simulink model "ATOM_simple_planning_simulator"  (R2026a)
settings: Solver=ode4  StopTime=50  FixedStep=0.01
StopFcn:
  | if exist('costmap_active','var') && ...
  |    exist('vehicle','var') && ...
  |    exist('parking_path','var') && ...
  |    ~isempty(parking_path)
  | 
  |     plotPlan(costmap_active, vehicle, parking_path);
  | else
  |     warning('No valid parking path is available for plotting.');
  | end
model workspace (MAT data in the model file):
  vehicle : object (value not decoded)
symbols that are objects in the model workspace (value not decoded): vehicle
undefined symbols (not defined in the file or in its folder): delta_f_LUT, gain4WS_LUT, k_ref_LUT, kappa_gain_BP, Ki, Kp, lateral, longitudinal, planning_validator, rr_gain_BP, rr_LUT, stanley, velocity_smoother
libraries: slpidlib x1, simulink x1
(part 5 of 7)

== matlab function ATOM_simple_planning_simulator/Plot vehicle/Plot vehicle Front reference frame ==
  settings: updateMethod=DISCRETE
  data: kinematic input Bus: KinematicStateBus; steer_front input double; steer_rear input double; veh input; traj input
function plotVehicleFront(kinematic, steer_front, steer_rear, veh, traj)

%% Vehicle parameters

L  = veh(3);
track = veh(4);

front_overhang = veh(5);
rear_overhang  = veh(6);
left_overhang = veh(7);
right_overhang = veh(8);

vehicle_length  = L + front_overhang + rear_overhang;
vehicle_width = track + left_overhang + right_overhang;

wheel_width = veh(2);
wheel_radius = veh(1);

%% Reference trajectory

x_ref = traj.pose.position.x;
y_ref = traj.pose.position.y;

yaw_ref = zeros(length(x_ref),1);


for i=1:length(x_ref)

    yaw_ref(i)=2*atan2(...
        traj.pose.orientation.qz(i),...
        traj.pose.orientation.qw(i));
end


%% Current kinematic state

x = kinematic.pose.position.x;
y = kinematic.pose.position.y;

qz = kinematic.pose.orientation.z;
qw = kinematic.pose.orientation.w;

yaw = 2*atan2(qz,qw);

vx = kinematic.twist.linear.x;

steer_front = steer_front;
steer_rear = steer_rear;

%% Position and orientation vehicle body

vehicle_body = [front_overhang vehicle_width/2;
                front_overhang -vehicle_width/2;
                -L-rear_overhang -vehicle_width/2;
                -L-rear_overhang vehicle_width/2;
                front_overhang vehicle_width/2];

R_body = [ cos(yaw) -sin(yaw)
    sin(yaw)  cos(yaw) ];

body_world = (R_body*vehicle_body')';

body_world(:,1)=body_world(:,1)+x;
body_world(:,2)=body_world(:,2)+y;


%% Position and orientation wheels

wheel_body = [wheel_radius  wheel_width/2
                wheel_radius -wheel_width/2
                -wheel_radius -wheel_width/2
                -wheel_radius  wheel_width/2
                wheel_radius  wheel_width/2];

FL = [0  track/2];
FR = [0 -track/2];
RL = [-L  track/2];
RR = [-L -track/2];

centers = [FL;
    FR;
    RL;
    RR];

centers = (R_body*centers')';

centers(:,1) = centers(:,1)+x;
centers(:,2) = centers(:,2)+y;

wheelFL = transformWheel(centers(1,:),steer_front,yaw,wheel_body);
wheelFR = transformWheel(centers(2,:),steer_front,yaw,wheel_body);
wheelRL = transformWheel(centers(3,:),steer_rear,yaw,wheel_body);
wheelRR = transformWheel(centers(4,:),steer_rear,yaw,wheel_body);



persistent hFig
persistent ax
persistent hBody
persistent hWheelFL
persistent hWheelFR
persistent hWheelRL
persistent hWheelRR
persistent hTrajectory
persistent TrajX
persistent TrajY
persistent hRefTraj 
persistent hArrow


if isempty(hBody)
    hFig = figure(13);
    clf

    ax = axes(hFig);

    hold(ax,'on')
    axis(ax,'equal')
    grid(ax,'on')


    xlabel(ax,'x [m]')
    ylabel(ax,'y [m]')

    hBody = plot(body_world(:,1),...
        body_world(:,2),...
        'k','LineWidth',2);

    hWheelFL = plot(wheelFL(:,1),...
        wheelFL(:,2),...
        'r','LineWidth',2);

    hWheelFR = plot(wheelFR(:,1),...
        wheelFR(:,2),...
        'r','LineWidth',2);

    hWheelRL = plot(wheelRL(:,1),...
        wheelRL(:,2),...
        'b','LineWidth',2);

    hWheelRR = plot(wheelRR(:,1),...
        wheelRR(:,2),...
        'b','LineWidth',2);

    TrajX = x;
    TrajY = y;

    hTrajectory = plot(TrajX,...
                       TrajY,...
                       'g','LineWidth',1);

    hRefTraj=plot(x_ref,y_ref,'b','LineWidth',2);

    step=5;

    hArrow=quiver(...
        x_ref(1:step:end),...
        y_ref(1:step:end),...
        cos(yaw_ref(1:step:end)),...
        sin(yaw_ref(1:step:end)),...
        0.5,...
        'r');

else

    set(hBody,...
        'XData',body_world(:,1),...
        'YData',body_world(:,2));

    set(hWheelFL,...
        'XData',wheelFL(:,1),...
        'YData',wheelFL(:,2));

    set(hWheelFR,...
        'XData',wheelFR(:,1),...
        'YData',wheelFR(:,2));

    set(hWheelRL,...
        'XData',wheelRL(:,1),...
        'YData',wheelRL(:,2));

    set(hWheelRR,...
        'XData',wheelRR(:,1),...
        'YData',wheelRR(:,2));

    TrajX(end+1) = x;
    TrajY(end+1) = y;

 
    set(hTrajectory,...
        'XData',TrajX,...
        'YData',TrajY);

    set(hRefTraj,...
        'XData',x_ref,...
        'YData',y_ref);

    

end

margin = 12;
xlim(ax, [x-margin x+margin])
ylim(ax, [y-margin y+margin])

% xlim([-20 20])
% ylim([-20 20])

drawnow limitrate
pause(0.01)


end

== matlab function ATOM_simple_planning_simulator/Plot vehicle/SetStanleyTrajectory/calcLongOffsetToSegment ==
  data: seg_idx input; ego_pose input; trajectory input Bus: TrajectoryDataBus; ego_offset_to_segment output
function ego_offset_to_segment = calcLongOffsetToSegment(seg_idx, ego_pose, trajectory)

ego_offset_to_segment = calcLongitudinalOffsetToSegment(trajectory, seg_idx, ego_pose);

end

== matlab function ATOM_simple_planning_simulator/Plot vehicle/SetStanleyTrajectory/findFirstNearestSegmentIndexWithSoftConstraints ==
  data: trajectory input; dist_threshold input; yaw_threshold input; nearest_seg_idx output; pose input
function nearest_seg_idx = findNearestSegmentIndexWithSoftConstraints( ...
    trajectory, dist_threshold, yaw_threshold, pose)


%% Step 1:
% Find nearest point index

nearest_idx = findFirstNearestIndexWithSoftConstraints( ...
    trajectory, ...
    pose, ...
    dist_threshold, ...
    yaw_threshold);


N = length(trajectory.pose.position.x);


%% Step 2:
% Convert point index into segment index

% First point
if nearest_idx == 1

    nearest_seg_idx = 1;
    return

end


% Last point
if nearest_idx == N

    nearest_seg_idx = N-1;
    return

end



%% Step 3:
% Determine whether ego lies before or after nearest point
%
% Equivalent to Autoware:
%
% signed_length =
% calcLongitudinalOffsetToSegment(points,
%                                 nearest_idx,
%                                 pose.position)


signed_length = calcLongitudinalOffsetToSegment( ...
    trajectory,...
    nearest_idx,...
    pose);



%% Step 4:
% Choose segment

if signed_length <= 0

    % ego is before nearest point
    %
    % Autoware:
    % return nearest_idx - 1;

    nearest_seg_idx = nearest_idx - 1;


else

    % ego is after nearest point
    %
    % Autoware:
    % return nearest_idx;

    nearest_seg_idx = nearest_idx;

end


end

== matlab function ATOM_simple_planning_simulator/Lateral run()/CalculateStanley/getData/calculate curvature predicted/CalcTrajectoryCurvature ==
  data: trajectory input Bus: TrajectoryDataBus; curvature output; nearest_idx input; idx_dist input
function curvature = ComputeNearestCurvature( ...
    trajectory,...
    nearest_idx, idx_dist)


%% ============================================================
% COMPUTE NEAREST TRAJECTORY CURVATURE
%
% Equivalent to:
%
% autoware::motion_utils::calcTrajectoryCurvatureFrom3Points()
%
% Difference:
%
% - Autoware computes curvature for the whole trajectory
% - Here only the curvature at nearest_idx is required
%   for Stanley controller
%
% Inputs:
%
% trajectory:
%   Reference trajectory
%
% nearest_idx:
%   Nearest trajectory point index
%
% idx_dist:
%   Distance in samples used for three-point fitting
%
%
% Output:
%
% curvature:
%   Local trajectory curvature [1/m]
%
% ============================================================

N = length(trajectory.pose.position.x);



%% Check trajectory length

if N < 3

    curvature = 0;
    return

end



%% Clamp index

nearest_idx = max(1,min(nearest_idx,N));



%% Select three points
%
% Equivalent to Autoware:
%
% p0 = trajectory[i-idx_dist]
% p1 = trajectory[i]
% p2 = trajectory[i+idx_dist]
%
% ============================================================


idx_prev = nearest_idx - min(idx_dist, nearest_idx-1);

idx_next = nearest_idx + min(idx_dist, N-nearest_idx);



p0 = [
    trajectory.pose.position.x(idx_prev),...
    trajectory.pose.position.y(idx_prev)
];


p1 = [
    trajectory.pose.position.x(nearest_idx),...
    trajectory.pose.position.y(nearest_idx)
];


p2 = [
    trajectory.pose.position.x(idx_next),...
    trajectory.pose.position.y(idx_next)
];



%% Compute curvature

curvature = calc_curvature(p0,p1,p2);


end

== matlab function ATOM_simple_planning_simulator/Lateral run()/CalculateStanley/getData/calculate curvature predicted/ComputeIdxDist ==
  data: points_interval input; idx_dist output; vel_smoother input
function idx_dist = ComputeIdxDist( ...
    points_interval, ...
    vel_smoother)

% ComputeIdxDist
%
% Computes the point offset used for trajectory curvature estimation.
%
% The curvature is evaluated using three trajectory points separated by a
% fixed physical distance. Since the trajectory is sampled with a constant
% spatial interval (points_interval), this function converts the desired
% curvature calculation distance into the corresponding point index offset.
%
% In other words, idx_dist represents the number of trajectory points
% corresponding to the specified curvature calculation distance.
%
% Equivalent to the Autoware implementation:
%
% idx_dist = max(int(curvature_calculation_distance / points_interval), 1);

curvature_calculation_distance = vel_smoother(1);

idx_dist = max( ...
    floor(curvature_calculation_distance / points_interval), ...
    1);

== matlab function ATOM_simple_planning_simulator/Lateral run()/CalculateStanley/getData/calculate curvature predicted/ComputePointsInterval ==
  data: input_points_interval input; vel_smoother input; use_resampling input; points_interval output
function points_interval = computePointsInterval(input_points_interval, ...
    vel_smoother, use_resampling)

% Compute the trajectory points interval used for preprocessing.
%
% If resampling is enabled, a constant spatial interval is imposed.
% Otherwise, the original trajectory point spacing is preserved.

sample_ds = vel_smoother(3,1);

if use_resampling

    points_interval = sample_ds;

else

    points_interval = input_points_interval;

end

end

== matlab function ATOM_simple_planning_simulator/Lateral run()/CalculateStanley/VerifyStanleyStatus ==
  data: steering_cmd input; stanley_solved_status output boolean; reason output
function [stanley_solved_status, reason] = VerifyStanleyStatus(steering_cmd)

% reason codes:
% 0 = OK
% 1 = Steering command is NaN/Inf
%
% Attention: in Autoware, reason is a String type. Just Simulink struggles
% with it.

stanley_solved_status = true;
reason = uint8(0);

if ~isfinite(steering_cmd)
    stanley_solved_status = false;
    reason = uint8(1);
end

== matlab function ATOM_simple_planning_simulator/Lateral run()/MATLAB Function1 ==
  data: solved input; previous_status output; reason input; previous_status input; previous_reason input; previous_reason output
function [previous_status, previous_reason] = StanleyStatusManager( ...
    solved,...
    reason,...
    previous_status,...
    previous_reason)

% ATTENTION!!!
% In Autoware, stanley_solved_status (originally mpc_solved_status) 
% is a struct, where equivalently:
% - solved = stanley_solved_status.result
% - reason = stanley_solved_status.reason
%
% StanleyStatusManager here is not implemented since it doesn't change the
% implementation of the controller.

previous_status = solved;
previous_reason = reason;

== matlab function ATOM_simple_planning_simulator/Parking Scenario/Costmap generation: perpendicular lot/Perpendicular Parking ==
  settings: updateMethod=DISCRETE
  data: veh input; costmap output Bus: OccupancyGridBus; start_pose output; goal_pose output
function [costmap, start_pose, goal_pose] = costmapPerpendicularLot(veh)
%COSTMAPPERPENDICULARLOT  Single row of 7 bays, one left empty at x = 0.
%
% Reproduces autoware_costmap_generator geometry:
%   grid_resolution 0.3, grid_length_x/y 70.0, expand_polygon_size 0.5
% The primitives layer is INVERTED: background occupied, lot carved out.

persistent occ

res = 0.3;   W = 234;   H = 234;
origin_x = -(W/2)*res;
origin_y = -(H/2)*res;

bay_x     = (-3:3)*3.6;      % 7 bays, 3.6 m pitch
bay_y     = 8.75;
empty_bay = 4;               % x = 0

if isempty(occ)
    [IX, IY] = meshgrid(0:W-1, 0:H-1);
    X = origin_x + IX*res;
    Y = origin_y + IY*res;

    lot_x = [-15  15  15 -15];
    lot_y = [-12 -12  12  12];
    occ = ones(H,W);
    occ(inpolygon(X, Y, lot_x, lot_y)) = 0;

    car_len = veh(5) + veh(3) + veh(6);
    car_wid = veh(4) + veh(7) + veh(8);
    expand  = 0.5;
    L = car_len + expand;
    D = car_wid + expand;

    for k = 1:7
        if k ~= empty_bay
            qx = [ D/2 -D/2 -D/2  D/2] + bay_x(k);
            qy = [ L/2  L/2 -L/2 -L/2] + bay_y;
            occ(inpolygon(X, Y, qx, qy)) = 1;
        end
    end
end

start_pose = [0, 0,    0];
goal_pose  = [0, 7.75, pi/2];

costmap.info.resolution           = res;
costmap.info.width                = uint32(W);
costmap.info.height               = uint32(H);
costmap.info.origin.position.x    = origin_x;
costmap.info.origin.position.y    = origin_y;
costmap.info.origin.position.z    = 0;
costmap.info.origin.orientation.x = 0;
costmap.info.origin.orientation.y = 0;
costmap.info.origin.orientation.z = 0;
costmap.info.origin.orientation.w = 1;
costmap.data                      = int8(occ*100);
end

== matlab function ATOM_simple_planning_simulator/Lateral run()/UpdateSteeringOffset ==
  settings: updateMethod=DISCRETE
  data: steering input; twist input Bus: TwistBus; wheel_base input; update_vel_threshold input; update_steer_threshold input; average_num input; offset_limit input; steering_offset output; veh input
function steering_offset = updateSteeringOffset( ...
    steering,...
    twist,...
    wheel_base,...
    update_vel_threshold,...
    update_steer_threshold,...
    average_num,...
    offset_limit, ...
    veh)


persistent offset_storage
persistent count
persistent current_offset

rear_steering_ratio = veh(29);

if isempty(offset_storage)

    offset_storage = zeros(average_num,1);
    count = 0;
    current_offset = 0;

end


%% Current vehicle state

vx = twist.linear.x;
yaw_rate = twist.angular.z;



%% Check if offset update is allowed

update_offset = ...
    abs(vx) > update_vel_threshold && ...
    abs(steering) < update_steer_threshold;



if update_offset


    %% Estimate steering from vehicle motion

    rear_steering = rear_steering_ratio * steering;

    steer_angle_est = atan( ...
        yaw_rate*wheel_base/vx + tan(rear_steering));



    %% Compute offset

    new_offset = steering - steer_angle_est;



    %% Circular buffer

    count = count + 1;


    if count <= average_num

        offset_storage(count) = new_offset;

    else

        % shift left

        offset_storage(1:end-1)=offset_storage(2:end);

        offset_storage(end)=new_offset;

    end



    %% Compute average

    valid_samples = min(count,average_num);

    current_offset = mean(offset_storage(1:valid_samples));


end



%% Saturation (Autoware getOffset)

steering_offset = min(max(current_offset,...
    -offset_limit),...
    offset_limit);

end

== matlab function ATOM_simple_planning_simulator/Lateral run()/CalculateStanley/getData/calcNearestPoseInterpStanley1 ==
  data: self_pose input Bus: KinematicStateBus; trajectory input Bus: TrajectoryDataBus; nearest_pose output Bus: PoseBusStanley; max_dist input; max_yaw input; nearest_idx output
function [nearest_pose,nearest_idx]  = calcNearestPoseInterpStanley( ...
    self_pose, ...
    trajectory, ...
    max_dist, ...
    max_yaw)


%% ============================================================
% CALC NEAREST POSE INTERPOLATION FOR STANLEY CONTROLLER
%
% Equivalent to:
%
% MPCUtils::calcNearestPoseInterp()
%
% Differences with MPC:
%
% - Input trajectory is directly Trajectory message
% - No MPCTrajectory conversion
% - No relative_time prediction
% - Reference is already transformed to FRONT AXLE
%
% The function returns the continuous closest pose of the
% front axle on the reference trajectory.
%
% ============================================================


N = length(trajectory.pose.position.x);



%% ============================================================
% Initialization for code generation
% ============================================================

nearest_pose = struct();

nearest_pose.position.x = 0;
nearest_pose.position.y = 0;
nearest_pose.orientation.x = 0;
nearest_pose.orientation.y = 0;
nearest_pose.orientation.z = 0;
nearest_pose.orientation.w = 0;

nearest_idx = 1;

% nearest_velocity = 0;



if N == 0

    return

end



%% ============================================================
% Step 1:
% Find nearest trajectory index
%
% Equivalent to:
%
% findFirstNearestIndexWithSoftConstraints()
%
% ============================================================


nearest_idx = findFirstNearestIndexWithSoftConstraints( ...
    trajectory,...
    self_pose,...
    max_dist,...
    max_yaw);



%% ============================================================
% Single point trajectory
%
% Equivalent Autoware:
%
% if traj.size()==1
%
% ============================================================


if N == 1

    nearest_pose.x = trajectory.pose.position.x(1);
    nearest_pose.y = trajectory.pose.position.y(1);

    nearest_pose.orientation.x = trajectory.pose.orientation.qx(1);
    nearest_pose.orientation.y = trajectory.pose.orientation.qy(1);
    nearest_pose.orientation.z = trajectory.pose.orientation.qz(1);
    nearest_pose.orientation.w = trajectory.pose.orientation.qw(1);

    % nearest_velocity = trajectory.longitudinal_velocity_mps(1);

    return

end



%% ============================================================
% Step 2:
% Determine interpolation segment
%
% Equivalent to:
%
% calcLongitudinalOffset()
%
% ============================================================


if nearest_idx == 1

    prev_idx = 1;
    next_idx = 2;


elseif nearest_idx == N

    prev_idx = N-1;
    next_idx = N;


else


    p_nearest = [
        trajectory.pose.position.x(nearest_idx)
        trajectory.pose.position.y(nearest_idx)
        ];


    p_next = [
        trajectory.pose.position.x(nearest_idx+1)
        trajectory.pose.position.y(nearest_idx+1)
        ];


    signed_length = calcLongitudinalOffset( ...
        p_nearest,...
        p_next,...
        [self_pose.pose.position.x self_pose.pose.position.y]');


    if signed_length <= 0

        prev_idx = nearest_idx-1;
        next_idx = nearest_idx;

    else

        prev_idx = nearest_idx;
        next_idx = nearest_idx+1;

    end

end



%% ============================================================
% Step 3:
% Linear interpolation
%
% Equivalent to:
%
% nearest_pose.position =
% (1-ratio)*prev + ratio*next
%
% ============================================================


p_prev = [
    trajectory.pose.position.x(prev_idx)
    trajectory.pose.position.y(prev_idx)
];


p_next = [
    trajectory.pose.position.x(next_idx)
    trajectory.pose.position.y(next_idx)
];



segment_length = norm(p_next-p_prev);



% avoid division by zero

if segment_length < 1e-5


    nearest_pose.position.x = trajectory.pose.position.x(nearest_idx);
    nearest_pose.position.y = trajectory.pose.position.y(nearest_idx);


    nearest_pose.orientation.x = trajectory.pose.orientation.qx(nearest_idx);
    nearest_pose.orientation.y = trajectory.pose.orientation.qy(nearest_idx);
    nearest_pose.orientation.z = trajectory.pose.orientation.qz(nearest_idx);
    nearest_pose.orientation.w = trajectory.pose.orientation.qw(nearest_idx);

    % nearest_velocity = trajectory.longitudinal_velocity_mps(nearest_idx);


    return

end



%% Projection of ego on segment

offset = calcLongitudinalOffset( ...
    p_prev,...
    p_next,...
    [self_pose.pose.position.x self_pose.pose.position.y]');


ratio = min(max(offset / segment_length,0),1);



%% Interpolated position

nearest_pose.position.x = ...
    (1-ratio)*p_prev(1)+ratio*p_next(1);


nearest_pose.position.y = ...
    (1-ratio)*p_prev(2)+ratio*p_next(2);



%% ============================================================
% Yaw interpolation
%
% Equivalent:
%
% normalize_radian()
%
% ============================================================


yaw_prev = QuaternionToYaw( ...
    trajectory.pose.orientation.qx(prev_idx),...
    trajectory.pose.orientation.qy(prev_idx),...
    trajectory.pose.orientation.qz(prev_idx),...
    trajectory.pose.orientation.qw(prev_idx));


yaw_next = QuaternionToYaw( ...
    trajectory.pose.orientation.qx(next_idx),...
    trajectory.pose.orientation.qy(next_idx),...
    trajectory.pose.orientation.qz(next_idx),...
    trajectory.pose.orientation.qw(next_idx));


yaw_error = wrapToPi(yaw_prev-yaw_next);


nearest_yaw = wrapToPi( ...
    yaw_next + (1-ratio)*yaw_error);

[qx,qy,qz,qw] = yawToQuaternion(nearest_yaw);

nearest_pose.orientation.x = qx;
nearest_pose.orientation.y = qy;
nearest_pose.orientation.z = qz;
nearest_pose.orientation.w = qw;



% %% ============================================================
% % Velocity interpolation
% %
% % Stanley adaptation:
% %
% % The velocity is used for:
% % - gain scheduling
% % - softening factor
% %
% % ============================================================
% 
% 
% v_prev = trajectory.longitudinal_velocity_mps(prev_idx);
% 
% v_next = trajectory.longitudinal_velocity_mps(next_idx);
% 
% 
% nearest_velocity = ...
%     (1-ratio)*v_prev + ratio*v_next;


end

== matlab function ATOM_simple_planning_simulator/Lateral run()/CalculateStanley/getData/calculate curvature current/CalcTrajectoryCurvature ==
  data: trajectory input Bus: TrajectoryDataBus; curvature output; nearest_idx input; idx_dist input
function curvature = ComputeNearestCurvature( ...
    trajectory,...
    nearest_idx, idx_dist)


%% ============================================================
% COMPUTE NEAREST TRAJECTORY CURVATURE
%
% Equivalent to:
%
% autoware::motion_utils::calcTrajectoryCurvatureFrom3Points()
%
% Difference:
%
% - Autoware computes curvature for the whole trajectory
% - Here only the curvature at nearest_idx is required
%   for Stanley controller
%
% Inputs:
%
% trajectory:
%   Reference trajectory
%
% nearest_idx:
%   Nearest trajectory point index
%
% idx_dist:
%   Distance in samples used for three-point fitting
%
%
% Output:
%
% curvature:
%   Local trajectory curvature [1/m]
%
% ============================================================

N = length(trajectory.pose.position.x);



%% Check trajectory length

if N < 3

    curvature = 0;
    return

end



%% Clamp index

nearest_idx = max(1,min(nearest_idx,N));



%% Select three points
%
% Equivalent to Autoware:
%
% p0 = trajectory[i-idx_dist]
% p1 = trajectory[i]
% p2 = trajectory[i+idx_dist]
%
% ============================================================


idx_prev = nearest_idx - min(idx_dist, nearest_idx-1);

idx_next = nearest_idx + min(idx_dist, N-nearest_idx);



p0 = [
    trajectory.pose.position.x(idx_prev),...
    trajectory.pose.position.y(idx_prev)
];


p1 = [
    trajectory.pose.position.x(nearest_idx),...
    trajectory.pose.position.y(nearest_idx)
];


p2 = [
    trajectory.pose.position.x(idx_next),...
    trajectory.pose.position.y(idx_next)
];



%% Compute curvature

curvature = calc_curvature(p0,p1,p2);


end

== matlab function ATOM_simple_planning_simulator/Lateral run()/CalculateStanley/getData/calculate curvature current/ComputeIdxDist ==
  data: points_interval input; idx_dist output; vel_smoother input
function idx_dist = ComputeIdxDist( ...
    points_interval, ...
    vel_smoother)

% ComputeIdxDist
%
% Computes the point offset used for trajectory curvature estimation.
%
% The curvature is evaluated using three trajectory points separated by a
% fixed physical distance. Since the trajectory is sampled with a constant
% spatial interval (points_interval), this function converts the desired
% curvature calculation distance into the corresponding point index offset.
%
% In other words, idx_dist represents the number of trajectory points
% corresponding to the specified curvature calculation distance.
%
% Equivalent to the Autoware implementation:
%
% idx_dist = max(int(curvature_calculation_distance / points_interval), 1);

curvature_calculation_distance = vel_smoother(1);

idx_dist = max( ...
    floor(curvature_calculation_distance / points_interval), ...
    1);

== matlab function ATOM_simple_planning_simulator/Lateral run()/CalculateStanley/getData/calculate curvature current/ComputePointsInterval ==
  data: input_points_interval input; vel_smoother input; use_resampling input; points_interval output
function points_interval = computePointsInterval(input_points_interval, ...
    vel_smoother, use_resampling)

% Compute the trajectory points interval used for preprocessing.
%
% If resampling is enabled, a constant spatial interval is imposed.
% Otherwise, the original trajectory point spacing is preserved.

sample_ds = vel_smoother(3,1);

if use_resampling

    points_interval = sample_ds;

else

    points_interval = input_points_interval;

end

end

== matlab function ATOM_simple_planning_simulator/Lateral run()/CalculateStanley/RearToFrontOdometry ==
  data: rear_pose input Bus: KinematicStateBus; front_pose_pred output Bus: KinematicStateBus; wheel_base input
function front_pose_pred = RearToFrontOdometryCurrent( ...
    rear_pose, ...
    wheel_base)

front_pose_pred = rear_pose;

% 1. Estrazione dello Yaw dall'orientamento (Quaternion -> Yaw)
qx = rear_pose.pose.orientation.x;
qy = rear_pose.pose.orientation.y;
qz = rear_pose.pose.orientation.z;
qw = rear_pose.pose.orientation.w;
yaw = QuaternionToYaw(qx, qy, qz, qw);

% 2. Calcolo della Posizione Attuale dell'Asse Anteriore (Mappa/World Frame)
x_front_now = rear_pose.pose.position.x + wheel_base * cos(yaw);
y_front_now = rear_pose.pose.position.y + wheel_base * sin(yaw);

% 3. Velocità dell'Asse Anteriore espresso nel Frame Veicolo (Body Frame)
v_x_body = rear_pose.twist.linear.x;
v_y_body = rear_pose.twist.linear.y + rear_pose.twist.angular.z * wheel_base;

% 4. Conversione delle Velocità dal Frame Veicolo (Body) al Frame Mappa (World)
% Ruotiamo il vettore velocità [v_x_body, v_y_body] dell'angolo yaw attuale:
v_x_world = v_x_body * cos(yaw) - v_y_body * sin(yaw);
v_y_world = v_x_body * sin(yaw) + v_y_body * cos(yaw);

% 5. PREDIZIONE TEMPORALE (Coordinate t + tau nel Frame Mappa)
front_pose_pred.pose.position.x = x_front_now;
front_pose_pred.pose.position.y = y_front_now;
front_pose_pred.pose.position.z = rear_pose.pose.position.z;

% 6. Aggiornamento delle velocità nel messaggio di output (Frame Veicolo)
front_pose_pred.twist.linear.x = v_x_body;
front_pose_pred.twist.linear.y = v_y_body;
front_pose_pred.twist.linear.z = rear_pose.twist.linear.z;

% 7. L'orientamento rimane lo stesso (o aggiornato con il pitch/roll se presente)
front_pose_pred.pose.orientation = rear_pose.pose.orientation;

end

== matlab function ATOM_simple_planning_simulator/Lateral run()/CalculateStanley/getData/ChooseCurvature ==
  data: curvature_pred input; curvature output; curvature_curr input
function curvature = ChooseCurvature(curvature_pred, curvature_curr)

% =========================================
%
% Left turns: curvature > 0
% Right turns: curvature < 0
%
% =========================================

curvature_max = sin(2*0.7)/(2*cos(-0.7));

if abs(curvature_pred) >= abs(curvature_curr)
    if abs(curvature_pred) >= curvature_max
        sign_k = sign(curvature_pred);
        curvature = sign_k*curvature_max;
    else
        curvature = curvature_pred;
    end
else
    if abs(curvature_curr) >= curvature_max
        sign_k = sign(curvature_curr);
        curvature = sign_k*curvature_max;
    else
        curvature = curvature_curr;
    end


end

== matlab function ATOM_simple_planning_simulator/Lateral run()/Adaptive d0 ==
  data: d0 output; tau_steer input
function d0 = ComputeAdaptived0(tau_steer)

% d0 is the distance ahead of the vehicle, necessary for prediction.
% It's independent from current vehicle speed.
% We've seen that with time_constant = 0.27 --> d0 = 0.3.

d0 = (0.3/0.27)*tau_steer;

end

== matlab function ATOM_simple_planning_simulator/Lane Follower Scenario/Demanded trajectory generation: Serpentine/Trajectory Generator: 90° left turn critical for 2WS ==
  data: x output; y output; z output; qx output; qy output; qz output; qw output; longitudinal_velocity_mps output; lateral_velocity_mps output; acceleration_mps2 output; heading_rate_rps output; front_wheel_angle_rad output; rear_wheel_angle_rad output
function [x,y,z,qx,qy,qz,qw,...
          longitudinal_velocity_mps,...
          lateral_velocity_mps,...
          acceleration_mps2,...
          heading_rate_rps,...
          front_wheel_angle_rad,...
          rear_wheel_angle_rad] = trajectoryGenerator

N = 100;

%% Geometry

R = 3;                  % Radius [m]

N1 = 20;                % First straight
N2 = 30;                % Left curve
N3 = 30;                % Right curve
N4 = 20;                % Final straight


%% Allocate outputs

x = zeros(N,1);
y = zeros(N,1);
z = zeros(N,1);

qx = zeros(N,1);
qy = zeros(N,1);
qz = zeros(N,1);
qw = zeros(N,1);

longitudinal_velocity_mps = 6/3.6 * ones(N,1);

lateral_velocity_mps = zeros(N,1);
acceleration_mps2 = zeros(N,1);
heading_rate_rps = zeros(N,1);

front_wheel_angle_rad = zeros(N,1);
rear_wheel_angle_rad = zeros(N,1);


%% ========================================================================
%% First straight
%% ========================================================================

L1 = 2;

for i = 1:N1

    t = (i-1)/(N1-1);

    x(i) = t*L1;
    y(i) = 0;

    yaw = 0;

    qz(i) = sin(yaw/2);
    qw(i) = cos(yaw/2);

end


%% ========================================================================
%% First curve (LEFT)
%% ========================================================================

center1_x = L1;
center1_y = R;

theta = linspace(-pi/2,0,N2);

for k = 1:N2

    i = N1 + k;

    x(i) = center1_x + R*cos(theta(k));
    y(i) = center1_y + R*sin(theta(k));

    yaw = theta(k) + pi/2;

    qz(i) = sin(yaw/2);
    qw(i) = cos(yaw/2);

end


%% ========================================================================
%% Second curve (RIGHT)
%% Tangent to the previous one
%% ========================================================================

x_join = x(N1+N2);
y_join = y(N1+N2);

center2_x = x_join + R;
center2_y = y_join;

theta = linspace(pi,pi/2,N3);

for k = 1:N3

    i = N1 + N2 + k;

    x(i) = center2_x + R*cos(theta(k));
    y(i) = center2_y + R*sin(theta(k));

    yaw = theta(k) - pi/2;

    qz(i) = sin(yaw/2);
    qw(i) = cos(yaw/2);

end


%% ========================================================================
%% Final straight
%% ========================================================================

L2 = 15;

x0 = x(N1+N2+N3);
y0 = y(N1+N2+N3);

for k = 1:N4

    i = N1 + N2 + N3 + k;

    t = k/N4;

    x(i) = x0 + t*L2;
    y(i) = y0;

    yaw = 0;

    qz(i) = sin(yaw/2);
    qw(i) = cos(yaw/2);

end

end

== matlab function ATOM_simple_planning_simulator/Lane Follower Scenario/Demanded trajectory generation: smooth Parabola/Smoothed Parabola trajectory ==
  data: x output double; y output double; z output double; qx output double; qy output double; qz output double; qw output double; longitudinal_velocity_mps output double; lateral_velocity_mps output; acceleration_mps2 output; heading_rate_rps output; front_wheel_angle_rad output; rear_wheel_angle_rad output
function [x,y,z,qx,qy,qz,qw,longitudinal_velocity_mps, lateral_velocity_mps, acceleration_mps2, heading_rate_rps, front_wheel_angle_rad, rear_wheel_angle_rad] ...
            = trajectoryGenerator

N=100;

L=50;
Yend=20;


x=zeros(N,1);
y=zeros(N,1);
z=zeros(N,1);


qx=zeros(N,1);
qy=zeros(N,1);
qz=zeros(N,1);
qw=zeros(N,1);

longitudinal_velocity_mps=zeros(N,1);
lateral_velocity_mps=zeros(N,1);
acceleration_mps2=zeros(N,1);
heading_rate_rps=zeros(N,1);
front_wheel_angle_rad=zeros(N,1);
rear_wheel_angle_rad=zeros(N,1);

for i=1:N

    s=(i-1)/(N-1)*L;

    x(i)=s;

    a=Yend/L^2;

    y(i)=a*s^2;

    yaw=atan(2*a*s);


    qx(i)=0;
    qy(i)=0;
    qz(i)=sin(yaw/2);
    qw(i)=cos(yaw/2);


    longitudinal_velocity_mps(i)=5;

end

== matlab function ATOM_simple_planning_simulator/LongitudinalRun()/nearest_idx ==
  data: trajectory input; nearest_idx output; self_pose input; max_dist input; max_yaw input
function nearest_idx = findFirstNearestIndexWithSoftConstraints(trajectory, self_pose, max_dist, max_yaw)

nearest_idx = findFirstNearestIndexWithSoftConstraints( ...
    trajectory,...
    self_pose,...
    max_dist,...
    max_yaw);

end

== matlab function ATOM_simple_planning_simulator/velocity_smoother_node/ApplyLateralAccelerationFilter - velocity_smoother node/ComputeVelocityProfile and Acceleration ==
  data: a_accel_max input; a_decel_max input; v_start input; v_end input; trajectory output; trajectory input Bus: TrajectoryDataBus
function trajectory = ComputeVelocityProfile( ...
    a_accel_max, a_decel_max, v_start, v_end, trajectory)
%% This function is mainly to calculate the longitudinal velocity and acceleration profile of
%%on the trajectory in order to be in the output trajectory bus of the velocity smoother block
%%going to the vehicle model

N  = length(trajectory.longitudinal_velocity_mps);
px = trajectory.pose.position.x;
py = trajectory.pose.position.y;

%% Pass 1: arc-length spacing between consecutive points
ds = zeros(N-1,1);
for i = 1:N-1
    ds(i) = sqrt( (px(i+1)-px(i))^2 + (py(i+1)-py(i))^2 );
end

%% Pass 2: backward - deceleration feasibility
% Answers: how fast can I be here and still slow down for what's ahead?
v_bwd    = trajectory.longitudinal_velocity_mps;   % ceiling from prior stages
v_bwd(N) = min(v_bwd(N), v_end);
for i = N-1:-1:1
    v_reach  = sqrt( v_bwd(i+1)^2 + 2*a_decel_max*ds(i) );
    v_bwd(i) = min( v_bwd(i), v_reach );
end

%% Pass 3: forward - acceleration feasibility
% Answers: how fast can I actually have gotten to here?
v    = v_bwd;
v(1) = min( v_bwd(1), v_start );
for i = 2:N
    v_reach = sqrt( v(i-1)^2 + 2*a_accel_max*ds(i-1) );
    v(i)    = min( v_bwd(i), v_reach );
end

%% Extract acceleration from the finished profile
a = zeros(N,1);
for i = 1:N-1
    if ds(i) > 1e-6
        a(i) = ( v(i+1)^2 - v(i)^2 ) / ( 2*ds(i) );
    else
        a(i) = 0;      % zero-length segment guard
    end
end
a(N) = 0;              % no segment ahead of the last point

trajectory.longitudinal_velocity_mps = v;
trajectory.acceleration_mps2         = a;
end

== matlab function ATOM_simple_planning_simulator/velocity_smoother_node/ApplyLateralAccelerationFilter - velocity_smoother node/MATLAB Function1 ==
  data: a_lat_max input; trajectory output; min_curve_velocity input; curvature input; trajectory input Bus: TrajectoryDataBus
function trajectory  = ApplyLateralAccelerationLimit( ...
    a_lat_max, min_curve_velocity, curvature, trajectory)
% Limits trajectory velocity so that lateral acceleration v^2/R
% never exceeds a_lat_max.
%
% Equivalent to SmootherBase::applyLateralAccelerationFilter() in Autoware,
% minus the decel_distance_before/after_curve ramps - those are unnecessary
% here because ComputeVelocityProfile's backward pass already produces the
% early ramp-down from first principles.

N = length(trajectory.longitudinal_velocity_mps);

for i = 1:N

    k = abs(curvature(i));
    delta_r = trajectory.rear_wheel_angle_rad(i);

    % Straight segment: no lateral constraint
    if k < 1e-6
        continue
    end
    %given a limit and a corner, what's the fastest you can go?
    % v_max such that v^2 * k <= a_lat_max
    v_lat_max = sqrt(a_lat_max*cos(delta_r)/ k);

    % Floor, so tight curves don't demand a crawl
    v_lat_max = max(v_lat_max, min_curve_velocity);

    % Can only lower the ceiling, never raise it
    trajectory.longitudinal_velocity_mps(i) = ...
        min(trajectory.longitudinal_velocity_mps(i), v_lat_max);
end
fprintf('kappa max %.4f | v ceiling [%.2f %.2f]\n', ...
    max(abs(curvature)), min(trajectory.longitudinal_velocity_mps), ...
    max(trajectory.longitudinal_velocity_mps));
end

== matlab function ATOM_simple_planning_simulator/Vehicle Model/localization//acceleration function ==
  data: state input Bus: VehicleInternalStateBus; accel output Bus: AccelerationBus; veh input
function accel = IntStateToAccelerationState(state,veh)

L = veh(3);

vx = state.vx;
ax = state.acc;

delta_f = state.steer_front;
delta_r = state.steer_rear;

yaw_rate = (vx/L)*(tan(delta_f)-tan(delta_r));

ay = vx*yaw_rate;

accel.acceleration.linear.x = ax;
accel.acceleration.linear.y = ay;
accel.acceleration.linear.z = 0;

accel.acceleration.angular.x = 0;
accel.acceleration.angular.y = 0;
accel.acceleration.angular.z = 0;

end

== matlab function ATOM_simple_planning_simulator/Vehicle Model/localization//kinematic_state function ==
  data: state input Bus: VehicleInternalStateBus; kinematic output Bus: KinematicStateBus; veh input
function kinematic = IntStateToKinematicState(state, veh)


%% Vehicle parameters

L = veh(3);


%% Current state

x = state.x;
y = state.y;
yaw = state.yaw;



% NOTE:
% vx is the longitudinal velocity expressed in the vehicle body frame
% (base_link located at the center of the rear axle).
% The vehicle speed magnitude is reconstructed as
%
%   v = vx / cos(delta_r)
%
% under the pure-rolling assumption (alpha_f = alpha_r = 0).

vx = state.vx;

steer_front = state.steer_front;
steer_rear  = state.steer_rear;


%% Pose

kinematic.pose.position.x = x;
kinematic.pose.position.y = y;
kinematic.pose.position.z = 0;


[qx,qy,qz,qw] = yawToQuaternion(yaw);

% quaternion from yaw only

kinematic.pose.orientation.x = qx;
kinematic.pose.orientation.y = qy;
kinematic.pose.orientation.z = qz;
kinematic.pose.orientation.w = qw;



%% Twist

% Body frame velocity

kinematic.twist.linear.x = vx;

kinematic.twist.linear.y = ...              % Modified for 4WS considering beta = steer_rear
    vx*tan(steer_rear);

kinematic.twist.linear.z = 0;



% Angular velocity

kinematic.twist.angular.x = 0;
kinematic.twist.angular.y = 0;

kinematic.twist.angular.z = ...
    (vx/L) * ...
    (tan(steer_front)-tan(steer_rear));


end

== matlab function ATOM_simple_planning_simulator/Parking Scenario/Costmap generation: corridor occupancy grid/MATLAB Function ==
  data: veh input; costmap output Bus: OccupancyGridBus; start_pose output; goal_pose output
function [costmap, start_pose, goal_pose] = costmapNarrowCorridor(veh) %#ok<INUSD>
%COSTMAPNARROWCORRIDOR  8 m wide corridor.
%
% The planner turns in 5.47 m and the car is 2.66 m wide with its margin,
% so this corridor allows driving through but not turning around.
% Default task is a straight transit, which succeeds.
%
% To make it the limit case, change goal_pose heading to -pi/2 - a U-turn.
% That is expected to FAIL with a 5.47 m radius, and it is exactly the
% case a tighter turning circle would change.

persistent occ

res = 0.3;   W = 234;   H = 234;
origin_x = -(W/2)*res;
origin_y = -(H/2)*res;

if isempty(occ)
    [IX, IY] = meshgrid(0:W-1, 0:H-1);
    X = origin_x + IX*res;
    Y = origin_y + IY*res;

    lot_x = [ -4   4   4  -4];
    lot_y = [-12 -12  12  12];
    occ = ones(H,W);
    occ(inpolygon(X, Y, lot_x, lot_y)) = 0;
end

start_pose = [0, -8, pi/2];
goal_pose  = [0,  6, pi/2];

costmap.info.resolution           = res;
costmap.info.width                = uint32(W);
costmap.info.height               = uint32(H);
costmap.info.origin.position.x    = origin_x;
costmap.info.origin.position.y    = origin_y;
costmap.info.origin.position.z    = 0;
costmap.info.origin.orientation.x = 0;
costmap.info.origin.orientation.y = 0;
costmap.info.origin.orientation.z = 0;
costmap.info.origin.orientation.w = 1;
costmap.data                      = int8(occ*100);
end

== matlab function ATOM_simple_planning_simulator/Parking Scenario/Costmap generation: parking scenario beside a lane/MATLAB Function ==
  settings: updateMethod=DISCRETE
  data: veh input; costmap output Bus: OccupancyGridBus; start_pose output; goal_pose output
function [costmap, start_pose, goal_pose] = costmapDoubleRowLot(veh)
%COSTMAPDOUBLEROWLOT  Two rows of bays with a realistic aisle between them.
%
% Harder than the single-row lot: the car must enter the bay from an 8.6 m
% aisle with a 5.47 m turning radius, so it cannot swing in with one arc.
%
% Reproduces autoware_costmap_generator geometry:
%   grid_resolution 0.3, grid_length_x/y 70.0, expand_polygon_size 0.5

persistent occ

res = 0.3;   W = 234;   H = 234;
origin_x = -(W/2)*res;
origin_y = -(H/2)*res;

bay_x   = (-2:2)*3.6;          % 5 bays per row, 3.6 m pitch
row_y   = 6.0;                 % rows at y = +6 and y = -6  -> 8.6 m aisle
free_bay = 3;                  % the empty one, top row (x = 0)

if isempty(occ)
    [IX, IY] = meshgrid(0:W-1, 0:H-1);
    X = origin_x + IX*res;
    Y = origin_y + IY*res;

    % the lot, carved out of the wall
    lot_x = [-12  12  12 -12];
    lot_y = [ -9  -9   9   9];
    occ = ones(H,W);
    occ(inpolygon(X, Y, lot_x, lot_y)) = 0;

    car_len = veh(5) + veh(3) + veh(6);
    car_wid = veh(4) + veh(7) + veh(8);
    expand  = 0.5;
    L = car_len + expand;
    D = car_wid + expand;

    for k = 1:5
        % top row, one bay left empty
        if k ~= free_bay
            qx = [ D/2 -D/2 -D/2  D/2] + bay_x(k);
            qy = [ L/2  L/2 -L/2 -L/2] + row_y;
            occ(inpolygon(X, Y, qx, qy)) = 1;
        end
        % bottom row, fully occupied
        qx = [ D/2 -D/2 -D/2  D/2] + bay_x(k);
        qy = [ L/2  L/2 -L/2 -L/2] - row_y;
        occ(inpolygon(X, Y, qx, qy)) = 1;
    end
end

% --- the poses that belong to this scene ---------------------------------
start_pose = [-8, 0, 0];                    % in the aisle, heading east
goal_pose  = [ 0, row_y , pi/2 + pi];       % nose-in, top row, x = 0

costmap.info.resolution           = res;
costmap.info.width                = uint32(W);
costmap.info.height               = uint32(H);
costmap.info.origin.position.x    = origin_x;
costmap.info.origin.position.y    = origin_y;
costmap.info.origin.position.z    = 0;
costmap.info.origin.orientation.x = 0;
costmap.info.origin.orientation.y = 0;
costmap.info.origin.orientation.z = 0;
costmap.info.origin.orientation.w = 1;
costmap.data                      = int8(occ*100);
end

== matlab function ATOM_simple_planning_simulator/Parking Scenario/Costmap generation: complex parking situation/MATLAB Function ==
  settings: updateMethod=DISCRETE
  data: veh input; costmap output Bus: OccupancyGridBus; start_pose output; goal_pose output
function [costmap, start_pose, goal_pose] = ...
    costmapRoadsideParallelParking(veh)
%COSTMAPROADSIDEPARALLELPARKING
% A straight road with one parallel parking slot on its upper side.
%
% veh is the numeric vehicle-parameter vector:
% veh(3) = wheelbase
% veh(4) = wheel tread
% veh(5) = front overhang
% veh(6) = rear overhang
% veh(7) = left overhang
% veh(8) = right overhang

persistent occ

%% Grid

res = 0.3;
W = 234;
H = 234;

origin_x = -(W/2)*res;
origin_y = -(H/2)*res;

%% Vehicle dimensions

wheelbase      = veh(3);
wheel_tread    = veh(4);
front_overhang = veh(5);
rear_overhang  = veh(6);
left_overhang  = veh(7);
right_overhang = veh(8);

car_len = front_overhang + wheelbase + rear_overhang;
car_wid = wheel_tread + left_overhang + right_overhang;

%% Parking-scene parameters

% Obstacle inflation, matching the costmap generator
expand = 0.5;

parked_car_len = car_len + expand;
parked_car_wid = car_wid + expand;

% Road boundaries
road_x_min = -14;
road_x_max =  14;
road_y_min = -2.2;
road_y_max =  2.2;

% Tight empty-slot length
% With the current ATOM dimensions, this gives about 0.4 m clearance
% at each end for the inflated ego footprint.
slot_extra_length = 1.3;%1.3
slot_length = car_len + slot_extra_length;
slot_center_x = 0;

% Parking strip beside the road
parking_strip_width = parked_car_wid + 0.6;
parking_y = road_y_max + parking_strip_width/2;
parking_y_max = road_y_max + parking_strip_width;

% Small separation between parked vehicles outside the empty slot
inter_car_gap = 0.3;

%% Generate the occupancy grid

if isempty(occ)

    [IX,IY] = meshgrid(0:W-1,0:H-1);

    X = origin_x + IX*res;
    Y = origin_y + IY*res;

    % Begin with the whole map occupied
    occ = ones(H,W);

    % Create the road and its parking strip
    free_x = [ ...
        road_x_min, road_x_max, ...
        road_x_max, road_x_min];

    free_y = [ ...
        road_y_min, road_y_min, ...
        parking_y_max, parking_y_max];

    occ(inpolygon(X,Y,free_x,free_y)) = 0;

    %% Parked-car positions

    % Distance from the slot centre to either adjacent car centre
    adjacent_offset = ...
        (slot_length + parked_car_len)/2;

    % Two cars on each side of the empty slot
    parked_car_x = [ ...
        -adjacent_offset - parked_car_len - inter_car_gap, ...
        -adjacent_offset, ...
         adjacent_offset, ...
         adjacent_offset + parked_car_len + inter_car_gap];

    %% Add the parked cars

    for k = 1:length(parked_car_x)

        car_x = parked_car_x(k);

        % The cars are parallel to the road:
        % length along x and width along y
        qx = [ ...
            -parked_car_len/2, ...
             parked_car_len/2, ...
             parked_car_len/2, ...
            -parked_car_len/2] + car_x;

        qy = [ ...
            -parked_car_wid/2, ...
            -parked_car_wid/2, ...
             parked_car_wid/2, ...
             parked_car_wid/2] + parking_y;

        occ(inpolygon(X,Y,qx,qy)) = 1;
    end
end

%% Starting pose

% Rear-axle centre, travelling east along the road
start_pose = [-10, 0, 0];

%% Goal pose

% The parking slot is defined using its geometric centre, but Autoware's
% vehicle pose is the rear-axle centre.
body_center_from_rear_axle = ...
    (wheelbase + front_overhang - rear_overhang)/2;

goal_pose = [ ...
    slot_center_x - body_center_from_rear_axle, ...
    parking_y, ...
    0];

%% Costmap message

costmap.info.resolution = res;
costmap.info.width      = uint32(W);
costmap.info.height     = uint32(H);

costmap.info.origin.position.x = origin_x;
costmap.info.origin.position.y = origin_y;
costmap.info.origin.position.z = 0;

costmap.info.origin.orientation.x = 0;
costmap.info.origin.orientation.y = 0;
costmap.info.origin.orientation.z = 0;
costmap.info.origin.orientation.w = 1;

costmap.data = int8(occ*100);

end

== matlab function ATOM_simple_planning_simulator/Parking Scenario/Costmap generation: obstacle/MATLAB Function ==
  settings: updateMethod=DISCRETE
  data: veh input; costmap output Bus: OccupancyGridBus; start_pose output; goal_pose output
function [costmap, start_pose, goal_pose] = costmapSingleObstacle(veh) %#ok<INUSD>
%COSTMAPSINGLEOBSTACLE  Open area with one obstacle blocking the direct route.
% Paste this function into the connected costmap MATLAB Function block.
% Poses refer to the rear-axle centre; headings are in radians.
% Keep the vehicle input so the existing Simulink connections still match.

% Fixed dimensions match the existing OccupancyGrid bus.
res = 0.2;
W = 234;
H = 234;
origin_x = -(W/2)*res;
origin_y = -(H/2)*res;

% Editable scene dimensions [m].
area_x_min = -14;
area_x_max =  14;
area_y_min =  -8;
area_y_max =   8;

obstacle_center_x = 0;
obstacle_center_y = 0;
obstacle_length = 3;  % Along x.
obstacle_width  = 5;  % Along y.

start_pose = [-8, 0, 0];
goal_pose  = [ 8, 0, 0];

% Rebuild each call so changes cannot leave an old persistent map active.
[IX, IY] = meshgrid(0:W-1, 0:H-1);
X = origin_x + IX*res;
Y = origin_y + IY*res;

% Outside the open area is occupied; inside is free.
occupied = ~(X >= area_x_min & X <= area_x_max & ...
             Y >= area_y_min & Y <= area_y_max);

% The physical obstacle is added without extra inflation. collisionCheck
% already includes the planner's vehicle-shape margin.
obstacle = abs(X-obstacle_center_x) <= obstacle_length/2 & ...
           abs(Y-obstacle_center_y) <= obstacle_width/2;
occupied = occupied | obstacle;

costmap.info.resolution = res;
costmap.info.width  = uint32(W);
costmap.info.height = uint32(H);

costmap.info.origin.position.x = origin_x;
costmap.info.origin.position.y = origin_y;
costmap.info.origin.position.z = 0;
costmap.info.origin.orientation.x = 0;
costmap.info.origin.orientation.y = 0;
costmap.info.origin.orientation.z = 0;
costmap.info.origin.orientation.w = 1;

% Preserve the existing H-by-W int8 bus payload: free=0, occupied=100.
costmap.data = int8(occupied) .* int8(100);
end
